simulink library "OverrideSignal"  (R2022b)
settings: Solver=VariableStepAuto  StartTime=0.0  StopTime=10.0  RelTol=1e-3
libraries: FeaturePath x1, RTC x1
settings Model: Creator=kl13806  LastModifiedBy=kl13806
settings SolverCC: AlgebraicLoopSolver=TrustRegion
settings DebuggingCC: UnconnectedInputMsg=warning  UnconnectedOutputMsg=warning  UnconnectedLineMsg=warning  SFMachineParentedDataDiag=warning
settings ModelReferenceCC: EnableRefExpFcnMdlSchedulingChecks=on
settings RTWCC: DLArmComputeVersion=19.05

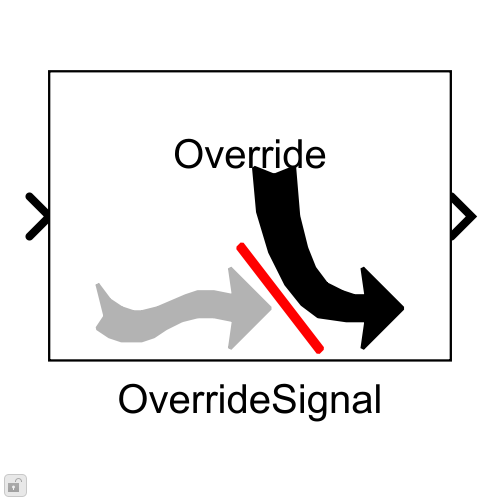
[thumbnail: Simulink's stored preview of the top-level diagram]
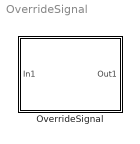
== system OverrideSignal ==
  OverrideSignal : Subsystem  mask(Bose Signal Override){MaskSignalName=, MaskDataTypeStr=single, MaskSignalWidth=1}
      mask prompts: MaskSignalName "Signal Name"; MaskDataTypeStr "Signal Type"; MaskSignalWidth "Signal Width"
      mask help: This creates the ability to override a signal at runtime. Only scalar and vector signals are currently supported (too lazy to put a reshaper block in there).
      settings: MoveFcn=SignalOverrideMask.CB_TriggerInit(gcbh);
      mask TypeOptions MaskSignalName: FeaturePath/FeatureName
      mask TypeOptions MaskDataTypeStr: RTC Override/REQElemType2 | RTC Override/RSPElemType2
      mask TypeOptions MaskSignalWidth: RTC Override/REQElemWidth2 | RTC Override/RSPElemWidth2
      mask Display:
      | [path,w,h] = IconOverrideSignalMask();
      | 
      | % work in pixels since the icon does not scale
      | pos = get(gcbh,'position');
      | bw = pos(3) - pos(1);
      | bh = pos(4) - pos(2);
      | 
      | % Draw centered icon
      | xAdj = bw/2 - w/2;
      | yAdj = 2; %bh/2 - h/2 + 4;
      | for i=1:length(path)
      |     if (path(i).rgb(1) >= 0)
      |         patch(path(i).x+xAdj, path(i).y+yAdj, path(i).rgb);
      |     end
      |     if (path(i).stroke(1) >= 0)
      |         plot(path(i).x+xAdj, path(i).y+yAdj);
      |     end
      | end
      | 
      | % Display some text
      | text(bw/2, bh-2,[MaskSignalName '\nOverride'], ...
      |     'horizontalAlignment','center', ...
      |     'VerticalAlignment','top');

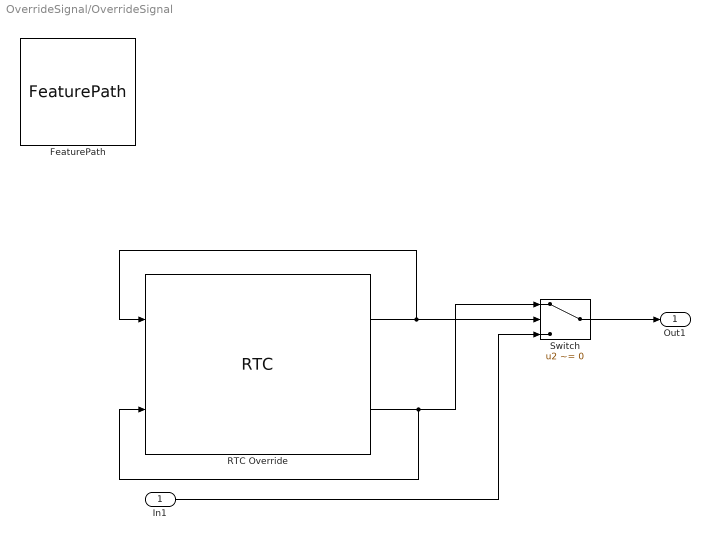
== system OverrideSignal/OverrideSignal ==
  In1 : Inport
  FeaturePath : FeaturePath/FeaturePath  IsGroup=off  GroupNumber=-1  IsModule=off  TriggerInit=[265 104 380 211]
  RTC Override : RTC/RTC  Description=Enables a signal to be overridden by a runtime request (RTC).  REQ_Priority=RTC_Mask.NormalPriority  RequestAtInit=off  EnableRequest=off  REQElemName1=enable_override  REQElemType1=uint32  REQElemWidth1=0  REQElemInitial1=0  REQElemName2=override_value  REQElemType2=single  REQElemWidth2=MaskSignalWidth  REQElemInitial2=[]  REQElemType3=uint32  REQElemWidth3=1  REQElemInitial3=[]  REQElemType4=uint32  REQElemWidth4=1  REQElemInitial4=[]  REQElemType5=uint32  REQElemWidth5=1  REQElemInitial5=[]  REQElemType6=uint32  REQElemWidth6=1  REQElemInitial6=[]  REQElemType7=uint32  REQElemWidth7=1  REQElemInitial7=[]  REQElemType8=uint32  REQElemWidth8=1  REQElemInitial8=[]  REQElemType9=uint32  REQElemWidth9=1  REQElemInitial9=[]  REQElemType10=uint32  REQElemWidth10=1  REQElemInitial10=[]  EnableResponse=on  EnableRSP_StatusIn=off  RSPElemName1=enable_override  RSPElemType1=uint32  RSPElemWidth1=1  RSPElemName2=override_value  RSPElemType2=single  RSPElemWidth2=MaskSignalWidth  RSPElemType3=uint32  RSPElemWidth3=1  RSPElemType4=uint32  RSPElemWidth4=1  RSPElemType5=uint32  RSPElemWidth5=1  RSPElemType6=uint32  RSPElemWidth6=1  RSPElemType7=uint32  RSPElemWidth7=1  RSPElemType8=uint32  RSPElemWidth8=1  RSPElemType9=uint32  RSPElemWidth9=1  RSPElemType10=uint32  RSPElemWidth10=1  EnableNotification=off  EnableNTF_PrepTrig=off  NTFElemType1=uint32  NTFElemWidth1=1  NTFElemType2=uint32  NTFElemWidth2=1  NTFElemType3=uint32  NTFElemWidth3=1  NTFElemType4=uint32  NTFElemWidth4=1  NTFElemType5=uint32  NTFElemWidth5=1  NTFElemType6=uint32  NTFElemWidth6=1  NTFElemType7=uint32  NTFElemWidth7=1  NTFElemType8=uint32  NTFElemWidth8=1  NTFElemType9=uint32  NTFElemWidth9=1  NTFElemType10=uint32  NTFElemWidth10=1  MaskMessageName=Override
  Switch : Switch  Criteria=u2 ~= 0  SaturateOnIntegerOverflow=off  InputSameDT=off
  Out1 : Outport  VectorParamsAs1DForOutWhenUnconnected=off
  wires:
  In1/1 -> Switch/3
  Switch/1 -> Out1/1
  RTC Override/2 -> RTC Override/2, Switch/1
  RTC Override/1 -> RTC Override/1, Switch/2
